simulink model "Cascade_Practice"  (R2024b)
settings: Solver=VariableStepAuto  StartTime=0.0  StopTime=10  RelTol=1e-3
libraries: slpidlib x1
settings Model: Creator=sh2323  LastModifiedBy=sh2323

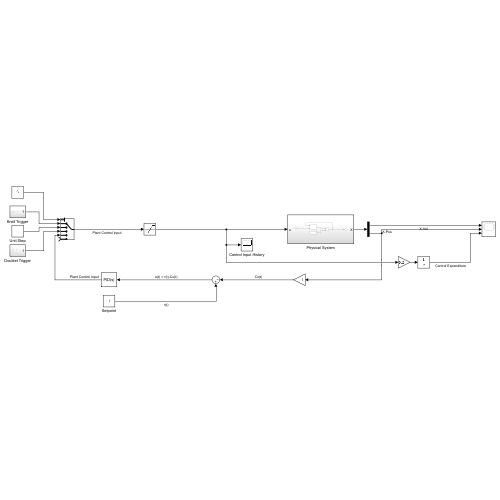
[thumbnail: Simulink's stored preview of the top-level diagram]
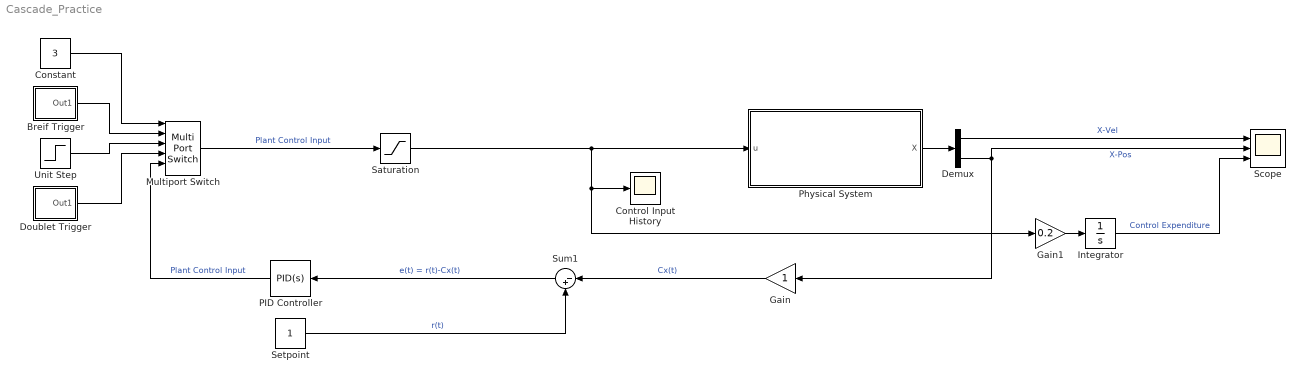
== system Cascade_Practice ==
  Breif Trigger : Subsystem
  Constant : Constant  Value=3
  Control Input History : Scope
  Demux : Demux  Outputs=2
  Doublet Trigger : Subsystem
  Gain : Gain
  Gain1 : Gain  Gain=0.2
  Integrator : Integrator
  Multiport Switch : MultiPortSwitch  DataPortOrder=Zero-based contiguous  Inputs=5  zeroidx=on  SaturateOnIntegerOverflow=off  InputSameDT=off
  PID Controller : slpidlib/PID Controller  Controller=PID  Form=Parallel  TimeDomain=Continuous-time  UseExternalTs=off  SampleTime=-1  IntegratorMethod=Forward Euler  FilterMethod=Forward Euler  ControllerParametersSource=internal  P=10.2948713552312  I=3.92722612104599  UseKiTs=off  D=6.45807028915118  UseExternalDerivativeSource=off  N=100  UseFilter=on  TunerSelectOption=Transfer Function Based (PID Tuner App)  InitialConditionSource=internal  InitialConditionForIntegrator=0  InitialConditionForFilter=0  DifferentiatorICPrevScaledInput=0  ExternalReset=none  TrackingMode=off  Kt=1  LimitOutput=off  SatLimitsSource=internal  UpperSaturationLimit=inf  LowerSaturationLimit=-inf  LinearizeAsGain=on  AntiWindupMode=none  Kb=1  LimitIntegrator=off  UpperIntegratorSaturationLimit=inf  LowerIntegratorSaturationLimit=-inf  POutMin=[]  POutMax=[]  IOutMin=[]  IOutMax=[]  DOutMin=[]  DOutMax=[]  NOutMin=[]  NOutMax=[]  SumOutMin=[]  SumOutMax=[]  SaturationOutMin=[]  SaturationOutMax=[]  PParamMin=[]  PParamMax=[]  IParamMin=[]  IParamMax=[]  DParamMin=[]  DParamMax=[]  NParamMin=[]  NParamMax=[]  KbParamMin=[]  KbParamMax=[]  KtParamMin=[]  KtParamMax=[]  KbOutMin=[]  KbOutMax=[]  KtOutMin=[]  KtOutMax=[]  IntegratorOutMin=[]  IntegratorOutMax=[]  FilterOutMin=[]  FilterOutMax=[]  SumI1OutMin=[]  SumI1OutMax=[]  SumI2OutMin=[]  SumI2OutMax=[]  SumI3OutMin=[]  SumI3OutMax=[]  SumI4OutMin=[]  SumI4OutMax=[]  SumDOutMin=[]  SumDOutMax=[]  DifferentiatorOutMin=[]  DifferentiatorOutMax=[]  FilterDiffOutCoefMin=[]  FilterDiffOutCoefMax=[]  ReciprocalOutMin=[]  ReciprocalOutMax=[]  SumDenOutMin=[]  SumDenOutMax=[]  SumNumOutMin=[]  SumNumOutMax=[]  DivideOutMin=[]  DivideOutMax=[]  UdiffTsProdOutMin=[]  UdiffTsProdOutMax=[]  NTsProdOutMin=[]  NTsProdOutMax=[]  UintegralTsProdOutMin=[]  UintegralTsProdOutMax=[]  UngainTsProdOutMin=[]  UngainTsProdOutMax=[]  ClampingZeroOutDataTypeStr=Inherit: Inherit via back propagation  ClampingZeroOutMin=[]  ClampingZeroOutMax=[]  FilterDenConstantOutDataTypeStr=Inherit: Inherit via back propagation  FilterDenConstantOutMin=[]  FilterDenConstantOutMax=[]  PCopyOutDataTypeStr=Inherit: Inherit via back propagation  PCopyOutMin=[]  PCopyOutMax=[]  NCopyOutDataTypeStr=Inherit: Inherit via back propagation  NCopyOutMin=[]  NCopyOutMax=[]  IntegratorContinuousStateAttributes=''  IntegratorStateMustResolveToSignalObject=off  IntegratorRTWStateStorageClass=Auto  FilterContinuousStateAttributes=''  FilterStateMustResolveToSignalObject=off  FilterRTWStateStorageClass=Auto  ParallelPVariant=InternalParameters  IdealPVariant=Disabled  IVariant=InternalParameters  DVariant=InternalParameters  IntegratorVariant=Continuous  SatVariant=Disabled  AWVariant=Passthrough  PCopyVariant=Disabled  TRVariant=Disabled  FdbkBlocksVariant=Forward  IdealPFdbkVariant=Disabled  SatFdbkVariant=Disabled  DerivativeFilterVariant=ContFilter  NVariant=InternalParameters  NCopyVariant=Disabled  FilterICVariant=InternalICsFilter  IntegratorICVariant=InternalICs  ExternalResetVariant=Disabled  TRSumVariant=Passthrough  SumFdbkVariant=Disabled  SumVariant=Sum_PID  TsampFilterVariant=InternalTs  TsampNgainVariant=Passthrough  TsampIntegralVariant=Disabled_SignalSpec  ExternalSaturationOutDataTypeStr=Inherit: Same as second input  DerivativeSourceVariant=ErrorSignal  PreIntVariant=InternalPreInt
  Physical System : Subsystem
  Saturation : Saturate  UpperLimit=2  LowerLimit=0
  Scope : Scope  NumInputPorts=3
  Setpoint : Constant
  Sum1 : Sum  Inputs=|-+
  Unit Step : Step  SampleTime=0
  wires:
  Constant/1 -> Multiport Switch/1
  Breif Trigger/1(Out1) -> Multiport Switch/2
  Unit Step/1 -> Multiport Switch/3
  Doublet Trigger/1(Out1) -> Multiport Switch/4
  Physical System/1(X) -> Demux/1
  Demux/2 -> Gain/1, Scope/2  "X-Pos"
  Demux/1 -> Scope/1  "X-Vel"
  Multiport Switch/1 -> Saturation/1  "Plant Control Input"
  PID Controller/1 -> Multiport Switch/5  "Plant Control Input"
  Setpoint/1 -> Sum1/2  "r(t)"
  Sum1/1 -> PID Controller/1  "e(t) = r(t)-Cx(t)"
  Gain/1 -> Sum1/1  "Cx(t)"
  Saturation/1 -> Gain1/1, Control Input History/1, Physical System/1(u)
  Integrator/1 -> Scope/3  "Control Expenditure"
  Gain1/1 -> Integrator/1

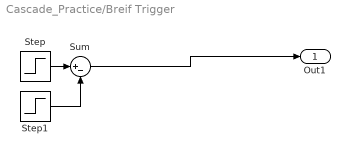
== system Cascade_Practice/Breif Trigger ==
  Step : Step  SampleTime=0
  Step1 : Step  Time=1.1  SampleTime=0
  Sum : Sum  Inputs=|+-
  Out1 : Outport
  wires:
  Step/1 -> Sum/1
  Step1/1 -> Sum/2
  Sum/1 -> Out1/1

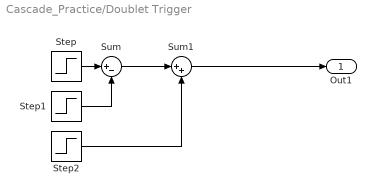
== system Cascade_Practice/Doublet Trigger ==
  Step : Step  SampleTime=0
  Step1 : Step  Time=1.1  After=2  SampleTime=0
  Step2 : Step  Time=1.2  SampleTime=0
  Sum : Sum  Inputs=|+-
  Sum1 : Sum  Inputs=|++
  Out1 : Outport
  wires:
  Step/1 -> Sum/1
  Step1/1 -> Sum/2
  Sum/1 -> Sum1/1
  Step2/1 -> Sum1/2
  Sum1/1 -> Out1/1

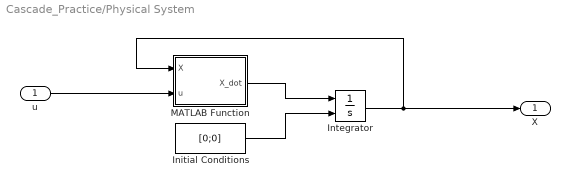
== system Cascade_Practice/Physical System ==
  u : Inport
  Initial Conditions : Constant  Value=[0;0]
  Integrator : Integrator  InitialConditionSource=external
  MATLAB Function : MATLAB Function  TreatAsAtomicUnit=on
  X : Outport
  wires:
  u/1 -> MATLAB Function/2(u)
  Integrator/1 -> X/1, MATLAB Function/1(X)
  MATLAB Function/1(X_dot) -> Integrator/1
  Initial Conditions/1 -> Integrator/2

== matlab function Cascade_Practice/Physical System/MATLAB Function ==
  data: X input size=2,1; u input size=1; X_dot output size=2,1
function X_dot = fcn(X,u)
%% Params:
m = 1;
c = -1;
k = -1;
d = 1;

%% EoM matrices
M = [m,0;0,1];
A = [c,k;1,0];
B = [d;0];

%  Mx_dot = Ax+Bu

X_dot = M\(A*X+B*u);
